simulink model "ctrl_ez"  (R2024b)
settings: configuration reference "CONFI" (kept outside this file)
InitFcn:
  | fidelity_pfc_vals;
  | wl=2*pi*50*150e-6;
  | 
  | gain_vac=1/(220*sqrt(2));
  | kpd = 5;
  | kpq = 5;
  | 
  | 
  | kid   =  1e2;
  | kiq   =  1e2;
  | 
  | kpvdc = .3;
  | kivdc =  .001;
values from neighbouring files (symbols this model uses):
  cos_th = cos(2*pi*50*t)    [fidelity_pfc_vals.m]
  sin_th = sin(2*pi*50*t)    [fidelity_pfc_vals.m]
  sin_th_vb = sin((2*pi*50*t)-(2*pi/3))    [fidelity_pfc_vals.m]
  sin_th_vc = sin((2*pi*50*t)+(2*pi/3))    [fidelity_pfc_vals.m]
  ts = 0.0001    [dic_pfc3ph.sldd]    (also in dictionary.sldd)
  tsw = 1/(fsw*1e3)    (= 1.53846153846e-05)    [fidelity_pfc_vals.m]
undefined symbols (not defined in the file or in its folder): DiscIntNeverNeededParam
libraries: mcbcontrolslib x18, simulink x5, dspswit3 x4, simulink_extras x2, slpidlib x2
(part 2 of 2)

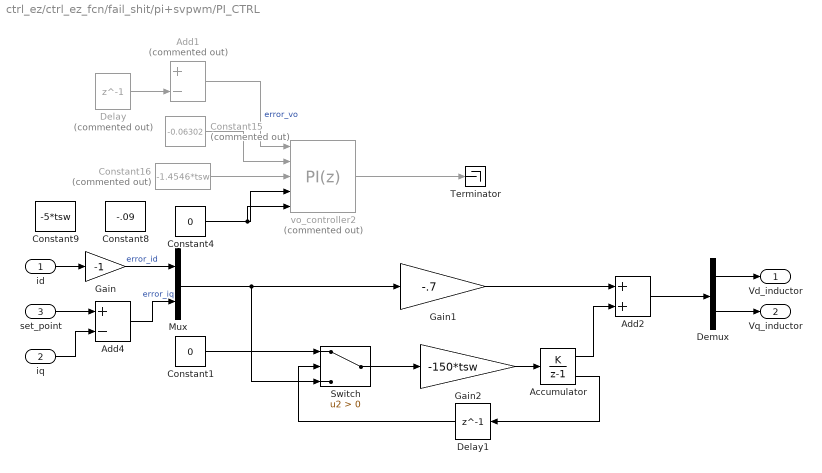
== system ctrl_ez/ctrl_ez_fcn/fail_shit/pi+svpwm/PI_CTRL ==
  id : Inport
  iq : Inport  Port=2  OutDataTypeStr=single
  set_point : Inport  Port=3
  Accumulator : DiscreteIntegrator  IntegratorMethod=Accumulation: Forward Euler  SampleTime=-1  LimitOutput=on  UpperSaturationLimit=50  LowerSaturationLimit=-50  ShowSaturationPort=on  ICPrevOutput=DiscIntNeverNeededParam  ICPrevScaledInput=DiscIntNeverNeededParam
  Add1 : Sum  Commented=on  Inputs=+-
  Add2 : Sum
  Add4 : Sum  Inputs=+-
  Constant1 : Constant  Value=0  OutDataTypeStr=single  SampleTime=-1
  Constant15 : Constant  Commented=on  Value=-0.06302  OutDataTypeStr=single  SampleTime=-1
  Constant16 : Constant  Commented=on  Value=-1.4546*tsw  OutDataTypeStr=single  SampleTime=-1
  Constant4 : Constant  Value=0  OutDataTypeStr=single  SampleTime=-1
  Constant8 : Constant  Value=-.09  OutDataTypeStr=single  SampleTime=-1
  Constant9 : Constant  Value=-5*tsw  OutDataTypeStr=single  SampleTime=-1
  Delay : Delay  Commented=on  DelayLength=1  InitialCondition=580
  Delay1 : Delay  DelayLength=1  InputProcessing=Columns as channels (frame based)
  Demux : Demux  Outputs=2
  Gain : Gain  Gain=-1  OutDataTypeStr=single
  Gain1 : Gain  Gain=-.7  OutDataTypeStr=single
  Gain2 : Gain  Gain=-150*tsw  OutDataTypeStr=single
  Mux : Mux  Inputs=2
  Switch : Switch  Criteria=u2 > Threshold  SaturateOnIntegerOverflow=off  InputSameDT=off
  Terminator : Terminator
  vo_controller2 : slpidlib/PID Controller  Commented=on  Controller=PI  Form=Parallel  TimeDomain=Discrete-time  UseExternalTs=on  SampleTime=-1  IntegratorMethod=Forward Euler  FilterMethod=Forward Euler  ControllerParametersSource=external  P=-0.053025  I=-1.4546  UseKiTs=on  D=0  UseExternalDerivativeSource=off  N=100  UseFilter=on  TunerSelectOption=Transfer Function Based (PID Tuner App)  InitialConditionSource=external  InitialConditionForIntegrator=0  InitialConditionForFilter=0  DifferentiatorICPrevScaledInput=0  ExternalReset=level  TrackingMode=off  Kt=1  LimitOutput=on  SatLimitsSource=internal  UpperSaturationLimit=300  LowerSaturationLimit=-300  LinearizeAsGain=on  AntiWindupMode=clamping  Kb=1  LimitIntegrator=off  UpperIntegratorSaturationLimit=inf  LowerIntegratorSaturationLimit=-inf  POutMin=[]  POutMax=[]  IOutMin=[]  IOutMax=[]  DOutMin=[]  DOutMax=[]  NOutMin=[]  NOutMax=[]  SumOutMin=[]  SumOutMax=[]  SaturationOutMin=[]  SaturationOutMax=[]  PParamMin=[]  PParamMax=[]  IParamMin=[]  IParamMax=[]  DParamMin=[]  DParamMax=[]  NParamMin=[]  NParamMax=[]  KbParamMin=[]  KbParamMax=[]  KtParamMin=[]  KtParamMax=[]  KbOutMin=[]  KbOutMax=[]  KtOutMin=[]  KtOutMax=[]  IntegratorOutMin=[]  IntegratorOutMax=[]  FilterOutMin=[]  FilterOutMax=[]  SumI1OutMin=[]  SumI1OutMax=[]  SumI2OutMin=[]  SumI2OutMax=[]  SumI3OutMin=[]  SumI3OutMax=[]  SumI4OutMin=[]  SumI4OutMax=[]  SumDOutMin=[]  SumDOutMax=[]  DifferentiatorOutMin=[]  DifferentiatorOutMax=[]  FilterDiffOutCoefMin=[]  FilterDiffOutCoefMax=[]  ReciprocalOutMin=[]  ReciprocalOutMax=[]  SumDenOutMin=[]  SumDenOutMax=[]  SumNumOutMin=[]  SumNumOutMax=[]  DivideOutMin=[]  DivideOutMax=[]  UdiffTsProdOutMin=[]  UdiffTsProdOutMax=[]  NTsProdOutMin=[]  NTsProdOutMax=[]  UintegralTsProdOutMin=[]  UintegralTsProdOutMax=[]  UngainTsProdOutMin=[]  UngainTsProdOutMax=[]  ClampingZeroOutDataTypeStr=Inherit: Inherit via back propagation  ClampingZeroOutMin=[]  ClampingZeroOutMax=[]  FilterDenConstantOutDataTypeStr=Inherit: Inherit via back propagation  FilterDenConstantOutMin=[]  FilterDenConstantOutMax=[]  PCopyOutDataTypeStr=Inherit: Inherit via back propagation  PCopyOutMin=[]  PCopyOutMax=[]  NCopyOutDataTypeStr=Inherit: Inherit via back propagation  NCopyOutMin=[]  NCopyOutMax=[]  IntegratorContinuousStateAttributes=''  IntegratorStateMustResolveToSignalObject=off  IntegratorRTWStateStorageClass=Auto  FilterContinuousStateAttributes=''  FilterStateMustResolveToSignalObject=off  FilterRTWStateStorageClass=Auto  ParallelPVariant=ExternalParameters  IdealPVariant=Disabled  IVariant=ExternalParameters  DVariant=Disabled  IntegratorVariant=Discrete  SatVariant=Enabled  AWVariant=DiscClampingParallel  PCopyVariant=Disabled  TRVariant=Disabled  FdbkBlocksVariant=Forward  IdealPFdbkVariant=Disabled  SatFdbkVariant=Disabled  DerivativeFilterVariant=Disabled  NVariant=Disabled  NCopyVariant=Disabled_SignalSpec  FilterICVariant=Disabled  IntegratorICVariant=ExternalICs  ExternalResetVariant=ExternalReset  TRSumVariant=Passthrough  SumFdbkVariant=Disabled  SumVariant=Sum_PI  TsampFilterVariant=InternalTs  TsampNgainVariant=Passthrough  TsampIntegralVariant=Passthrough  ExternalSaturationOutDataTypeStr=Inherit: Same as second input  DerivativeSourceVariant=Disabled  PreIntVariant=InternalPreInt
  Vd_inductor : Outport
  Vq_inductor : Outport  Port=2
  wires:
  Delay/1 -> Add1/2
  id/1 -> Gain/1
  Gain1/1 -> Add2/1
  set_point/1 -> Add4/1
  iq/1 -> Add4/2
  Demux/1 -> Vd_inductor/1
  Add1/1 -> vo_controller2/1  "error_vo"
  Add4/1 -> Mux/2  "error_iq"
  Add2/1 -> Demux/1
  Gain/1 -> Mux/1  "error_id"
  Constant15/1 -> vo_controller2/2
  Constant16/1 -> vo_controller2/3
  Mux/1 -> Switch/3, Gain1/1
  Constant1/1 -> Switch/1
  vo_controller2/1 -> Terminator/1
  Switch/1 -> Gain2/1
  Delay1/1 -> Switch/2
  Gain2/1 -> Accumulator/1
  Accumulator/1 -> Add2/2
  Accumulator/2 -> Delay1/1
  Demux/2 -> Vq_inductor/1
  Constant4/1 -> vo_controller2/4, vo_controller2/5

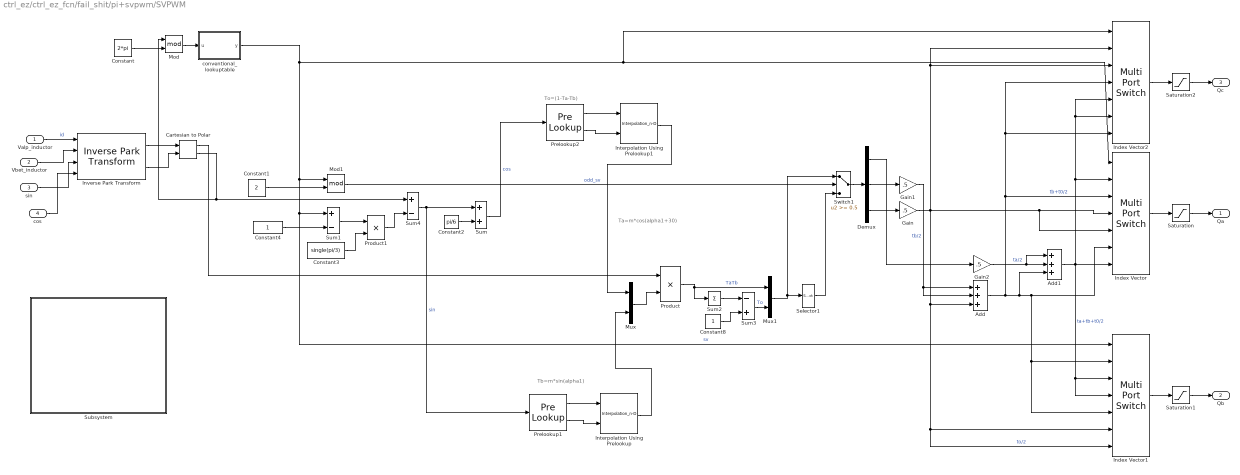
== system ctrl_ez/ctrl_ez_fcn/fail_shit/pi+svpwm/SVPWM ==
  note: Tb=m*sin(alpha1)
  note: Ta=m*cos(alpha1+30)
  note: To=(1-Ta-Tb)
  Valp_inductor : Inport
  Vbet_inductor : Inport  Port=2
  sin : Inport  Port=3
  cos : Inport  Port=4
  Add : Sum  Inputs=+++
  Add1 : Sum  Inputs=+++
  Cartesian to Polar : simulink_extras/Transformations/Cartesian to Polar
  Constant : Constant  Value=2*pi  OutDataTypeStr=single  SampleTime=-1
  Constant1 : Constant  Value=2  OutDataTypeStr=single  SampleTime=-1
  Constant2 : Constant  Value=pi/6  OutDataTypeStr=single  SampleTime=-1
  Constant3 : Constant  Value=single(pi/3)  VectorParams1D=off  OutDataTypeStr=single  SampleTime=-1
  Constant4 : Constant  VectorParams1D=off  OutDataTypeStr=single  SampleTime=-1
  Constant8 : Constant  OutDataTypeStr=single  SampleTime=-1
  Demux : Demux  Outputs=3
  Gain : Gain  Gain=.5  OutDataTypeStr=single
  Gain1 : Gain  Gain=.5  OutDataTypeStr=single
  Gain2 : Gain  Gain=.5  OutDataTypeStr=single
  Index Vector : MultiPortSwitch  Inputs=6  DiagnosticForDefault=None  SaturateOnIntegerOverflow=off  InputSameDT=off
  Index Vector1 : MultiPortSwitch  Inputs=6  DiagnosticForDefault=None  SaturateOnIntegerOverflow=off  InputSameDT=off
  Index Vector2 : MultiPortSwitch  Inputs=6  DiagnosticForDefault=None  SaturateOnIntegerOverflow=off  InputSameDT=off
  Interpolation Using Prelookup : Interpolation_n-D  NumberOfTableDimensions=1  Table=single(sin(0:2*pi/1024:2*pi))  InterpMethod=Flat  RemoveProtectionIndex=on  ValidIndexMayReachLast=on  InternalRulePriority=Speed
      settings: InputPortMap=u0,u1
  Interpolation Using Prelookup1 : Interpolation_n-D  NumberOfTableDimensions=1  Table=single(cos(0:2*pi/1024:2*pi))  InterpMethod=Flat  RemoveProtectionIndex=on  ValidIndexMayReachLast=on  InternalRulePriority=Speed
      settings: InputPortMap=u0,u1
  Inverse Park Transform : mcbcontrolslib/Inverse Park Transform  PhaseInput=Two inputs  AxisAlignment=D-axis  ThetaInput=Sine and Cosine electrical position  AngleInput=Per-unit  N_points=1024
      settings: LibrarySourceBlock=mcbhdllib/Controls/Math Transforms/Inverse Park Transform
  Mod : Math  Operator=mod
  Mod1 : Math  Operator=mod
  Mux : Mux  Inputs=2
  Mux1 : Mux  Inputs=2
  Prelookup1 : PreLookup  BreakpointsData=single((0:2*pi/1024:2*pi))  IndexSearchMethod=Evenly spaced points  BeginIndexSearchUsingPreviousIndexResult=on  UseLastBreakpoint=on
  Prelookup2 : PreLookup  BreakpointsData=single((0:2*pi/1024:2*pi))  IndexSearchMethod=Evenly spaced points  BeginIndexSearchUsingPreviousIndexResult=on  UseLastBreakpoint=on
  Product : Product  SaturateOnIntegerOverflow=on  OutDataTypeStr=Inherit: Same as first input
  Product1 : Product  OutDataTypeStr=single
  Saturation : Saturate  UpperLimit=.98  LowerLimit=.03
  Saturation1 : Saturate  UpperLimit=.98  LowerLimit=.03
  Saturation2 : Saturate  UpperLimit=.98  LowerLimit=.03
  Selector1 : Selector  InputPortWidth=3  IndexOptions=Index vector (dialog)  Indices=[2 1 3]  OutputSizes=1
  Subsystem : Subsystem
  Sum : Sum  SaturateOnIntegerOverflow=on
  Sum1 : Sum  Inputs=+-  OutDataTypeStr=single  AccumDataTypeStr=single
  Sum2 : Sum  Inputs=1  SaturateOnIntegerOverflow=on
  Sum3 : Sum  Inputs=-+  SaturateOnIntegerOverflow=on
  Sum4 : Sum  Inputs=+-  SaturateOnIntegerOverflow=on
  Switch1 : Switch  Threshold=0.5  InputSameDT=off
  conventional_lookuptable : MATLAB Function  TreatAsAtomicUnit=on
  Qa : Outport
  Qb : Outport  Port=2
  Qc : Outport  Port=3
  wires:
  Cartesian to Polar/2 -> Mod/1, Sum4/1
  Demux/2 -> Gain1/1
  Constant/1 -> Mod/2
  Gain1/1 -> Add/1, Add/2  "tb/2"
  Cartesian to Polar/1 -> Product/1
  Constant1/1 -> Mod1/2
  conventional_lookuptable/1(y) -> Index Vector1/1, Sum1/1, Mod1/1, Index Vector2/1, Index Vector/1  "sv"
  Constant4/1 -> Sum1/2
  Mod1/1 -> Switch1/2  "odd_sv"
  Constant3/1 -> Product1/2
  Constant2/1 -> Sum/2
  Demux/1 -> Gain2/1
  Sum4/1 -> Prelookup1/1, Sum/1  "sin"
  Sum/1 -> Prelookup2/1  "cos"
  Mux/1 -> Product/2
  Product/1 -> Mux1/1, Sum2/1  "TaTb"
  Sum2/1 -> Sum3/1
  Constant8/1 -> Sum3/2
  Sum3/1 -> Mux1/2  "To"
  Mux1/1 -> Switch1/1, Selector1/1
  Selector1/1 -> Switch1/3
  Switch1/1 -> Demux/1
  Demux/3 -> Gain/1
  Gain/1 -> Index Vector1/7, Index Vector1/6, Add/3, Index Vector/5, Index Vector/4, Index Vector2/3, Index Vector2/2  "to/2"
  Gain2/1 -> Add1/1, Add1/2  "ta/2"
  Add/1 -> Index Vector1/5, Index Vector1/2, Index Vector/6, Add1/3, Index Vector2/4, Index Vector2/7, Index Vector/3  "tb+t0/2"
  Add1/1 -> Index Vector1/4, Index Vector1/3, Index Vector2/5, Index Vector2/6, Index Vector/2, Index Vector/7  "ta+tb+t0/2"
  Mod/1 -> conventional_lookuptable/1(u)
  Prelookup1/1 -> Interpolation Using Prelookup/1
  Prelookup1/2 -> Interpolation Using Prelookup/2
  Prelookup2/2 -> Interpolation Using Prelookup1/2
  Prelookup2/1 -> Interpolation Using Prelookup1/1
  Interpolation Using Prelookup/1 -> Mux/2
  Interpolation Using Prelookup1/1 -> Mux/1
  Sum1/1 -> Product1/1
  Index Vector2/1 -> Saturation2/1
  Index Vector/1 -> Saturation/1
  Index Vector1/1 -> Saturation1/1
  Product1/1 -> Sum4/2
  Saturation2/1 -> Qc/1
  Saturation/1 -> Qa/1
  Saturation1/1 -> Qb/1
  Valp_inductor/1 -> Inverse Park Transform/1  "id"
  Vbet_inductor/1 -> Inverse Park Transform/2
  Inverse Park Transform/2 -> Cartesian to Polar/2
  Inverse Park Transform/1 -> Cartesian to Polar/1
  sin/1 -> Inverse Park Transform/3
  cos/1 -> Inverse Park Transform/4

== system ctrl_ez/ctrl_ez_fcn/fail_shit/pi+svpwm/clarke_park_tf ==
  a : Inport
  b : Inport  Port=2
  c : Inport  Port=3
  sin : Inport  Port=4
  cos : Inport  Port=5
  Clarke Transform : mcbcontrolslib/Clarke Transform  VariantControl=Variant2  PhaseInput=Three inputs  EnPowerInv=off
      settings: LibrarySourceBlock=mcbhdllib/Controls/Math Transforms/Clarke Transform
  Demux : Demux  Outputs=3
  Mux : Mux  Inputs=3
  Park Transform : mcbcontrolslib/Park Transform  PhaseInput=Two inputs  AxisAlignment=D-axis  ThetaInput=Sine and Cosine electrical position  AngleInput=Per-unit  N_points=1024
      settings: LibrarySourceBlock=mcbhdllib/Controls/Math Transforms/Park Transform
  Terminator : Terminator
  id : Outport
  iq : Outport  Port=2
  wires:
  a/1 -> Mux/1
  b/1 -> Mux/2
  c/1 -> Mux/3
  Mux/1 -> Clarke Transform/1
  Clarke Transform/1 -> Demux/1
  Demux/1 -> Park Transform/1
  Demux/3 -> Terminator/1
  Demux/2 -> Park Transform/2
  cos/1 -> Park Transform/4
  sin/1 -> Park Transform/3
  Park Transform/1 -> id/1
  Park Transform/2 -> iq/1

== system ctrl_ez/ctrl_ez_fcn/fail_shit/pi+svpwm/svm ==
  note: (Vmin+Vmax)/2
  In1 : Inport
  In2 : Inport  Port=2
  In3 : Inport  Port=3
  Add : Sum  Inputs=+-  RndMeth=Simplest  OutDataTypeStr=Inherit: Same as first input
  Add1 : Sum  Inputs=+-  RndMeth=Simplest  OutDataTypeStr=Inherit: Same as first input
  Add2 : Sum  RndMeth=Simplest  OutDataTypeStr=Inherit: Same as first input
  Add3 : Sum  RndMeth=Simplest  OutDataTypeStr=Inherit: Same as first input
  Add4 : Sum  RndMeth=Simplest  OutDataTypeStr=Inherit: Same as first input
  Add5 : Sum  Inputs=+-  RndMeth=Simplest  OutDataTypeStr=Inherit: Same as first input
  Demux : Demux  Outputs=3
  Demux1 : Demux  Outputs=3
  Demux2 : Demux  Outputs=3
  Gain : Gain  Gain=2/sqrt(3)  RndMeth=Simplest  OutDataTypeStr=Inherit: Same as input  ParamDataTypeStr=Inherit: Same as input
  Max : MinMax  Function=max  Inputs=3  RndMeth=Simplest  OutDataTypeStr=Inherit: Same as first input
  Min : MinMax  Inputs=3  RndMeth=Simplest  OutDataTypeStr=Inherit: Same as first input
  Min1 : MinMax  Inputs=3  RndMeth=Simplest  OutDataTypeStr=Inherit: Same as first input
  Mux2 : Mux  Inputs=3
  one_by_two : Gain  Gain=.5  RndMeth=Simplest  OutDataTypeStr=Inherit: Same as input  ParamDataTypeStr=Inherit: Same as input
  Out1 : Outport
  wires:
  Gain/1 -> Out1/1
  Add5/1 -> Add3/1, Add4/2, Add2/2
  Demux1/2 -> Add2/1, Min1/2
  Add3/1 -> Mux2/3
  Mux2/1 -> Gain/1
  Demux1/1 -> Add4/1, Min1/3
  Add2/1 -> Mux2/2
  Add4/1 -> Mux2/1
  Demux1/3 -> Min1/1, Add3/2
  Add/1 -> Add1/2  "vmx-vmn"
  Demux/3 -> Max/3
  Demux2/2 -> Min/2
  Demux/2 -> Max/2
  Demux/1 -> Max/1
  Demux2/1 -> Min/1
  Min/1 -> Add/2
  Max/1 -> Add/1
  Demux2/3 -> Min/3
  In1/1 -> Demux2/1, Demux/1, Demux1/1
  Add1/1 -> one_by_two/1  "vdc-vmx+mn"
  In2/1 -> Add1/1
  one_by_two/1 -> Add5/1
  Min1/1 -> Add5/2

== system ctrl_ez/ctrl_ez_fcn/fail_shit/pi+svpwm1/I_SET_PI_CTRL ==
  v_dc_error : Inport  OutDataTypeStr=single
  Accumulator : DiscreteIntegrator  IntegratorMethod=Accumulation: Forward Euler  SampleTime=-1  LimitOutput=on  UpperSaturationLimit=50  LowerSaturationLimit=-50  ShowSaturationPort=on  ICPrevOutput=DiscIntNeverNeededParam  ICPrevScaledInput=DiscIntNeverNeededParam
  Add2 : Sum
  Constant1 : Constant  Value=0  OutDataTypeStr=single  SampleTime=-1
  Delay1 : Delay  DelayLength=1  InputProcessing=Columns as channels (frame based)
  Gain1 : Gain  Gain=1/30  OutDataTypeStr=single
  Gain2 : Gain  Gain=0  OutDataTypeStr=single
  Saturation : Saturate  UpperLimit=30  LowerLimit=-30
  Switch : Switch  Criteria=u2 > Threshold  SaturateOnIntegerOverflow=off  InputSameDT=off
  i_set : Outport
  wires:
  Add2/1 -> Saturation/1
  Gain2/1 -> Accumulator/1
  Gain1/1 -> Add2/1
  Delay1/1 -> Switch/2
  Switch/1 -> Gain2/1
  Constant1/1 -> Switch/1
  Accumulator/1 -> Add2/2
  Accumulator/2 -> Delay1/1
  v_dc_error/1 -> Switch/3, Gain1/1  "error"
  Saturation/1 -> i_set/1

== system ctrl_ez/ctrl_ez_fcn/fail_shit/pi+svpwm1/PI_CTRL ==
  i_error : Inport  OutDataTypeStr=single
  Accumulator : DiscreteIntegrator  IntegratorMethod=Accumulation: Forward Euler  SampleTime=-1  LimitOutput=on  UpperSaturationLimit=50  LowerSaturationLimit=-50  ShowSaturationPort=on  ICPrevOutput=DiscIntNeverNeededParam  ICPrevScaledInput=DiscIntNeverNeededParam
  Add2 : Sum
  Constant1 : Constant  Value=0  OutDataTypeStr=single  SampleTime=-1
  Delay1 : Delay  DelayLength=1  InputProcessing=Columns as channels (frame based)
  Gain1 : Gain  Gain=100  OutDataTypeStr=single
  Gain2 : Gain  Gain=0  OutDataTypeStr=single
  Saturation : Saturate  Commented=through  UpperLimit=300  LowerLimit=-300
  Switch : Switch  Criteria=u2 > Threshold  SaturateOnIntegerOverflow=off  InputSameDT=off
  v_ind : Outport
  wires:
  i_error/1 -> Gain1/1, Switch/3  "error"
  Accumulator/2 -> Delay1/1
  Accumulator/1 -> Add2/2
  Constant1/1 -> Switch/1
  Switch/1 -> Gain2/1
  Delay1/1 -> Switch/2
  Gain1/1 -> Add2/1
  Gain2/1 -> Accumulator/1
  Add2/1 -> Saturation/1
  Saturation/1 -> v_ind/1

== system ctrl_ez/ctrl_ez_fcn/fail_shit/pi+svpwm1/Subsystem ==
  Constant : Constant  Value=0  SampleTime=-1
  Counter : dspswit3/Counter  Direction=Up  CountEvent=Free running  CounterSize=User defined  MaxCount=length(t)  InitialCount=0  Output=Count  HitValue=32  ResetInput=on  SamplesPerFrame=1  Ts=-1  CntDtype=uint32  HitDtype=Logical
  va_lt : LookupNDDirect  NumberOfTableDimensions=1  Table=single(sin_th*230*sqrt(2));  RemoveProtectionInput=on  TableDataTypeStr=single
  vb_lt : LookupNDDirect  NumberOfTableDimensions=1  Table=single(sin_th_vb*230*sqrt(2));  RemoveProtectionInput=on  TableDataTypeStr=single
  vc_lt : LookupNDDirect  NumberOfTableDimensions=1  Table=single(sin_th_vc*230*sqrt(2));  RemoveProtectionInput=on  TableDataTypeStr=single
  angle_wt : Outport
  angle_wt1 : Outport  Port=2
  angle_wt2 : Outport  Port=3
  wires:
  vc_lt/1 -> angle_wt2/1  "angle_wt"
  Counter/1 -> va_lt/1, vc_lt/1, vb_lt/1  "cnt"
  vb_lt/1 -> angle_wt1/1  "angle_wt"
  Constant/1 -> Counter/1
  va_lt/1 -> angle_wt/1  "angle_wt"

== system ctrl_ez/ctrl_ez_fcn/pll/dummy_pll/zcd ==
  v_ac : Inport  OutDataTypeStr=single
  AND : Logic  Inputs=4  AllPortsSameDT=off  OutDataTypeStr=boolean
  Compare To Zero : simulink/Logic and Bit Operations/Compare To Zero  relop=<  OutDataTypeStr=boolean
  Compare To Zero1 : simulink/Logic and Bit Operations/Compare To Zero  relop=<  OutDataTypeStr=boolean
  Compare To Zero2 : simulink/Logic and Bit Operations/Compare To Zero  relop=>  OutDataTypeStr=boolean
  Compare To Zero3 : simulink/Logic and Bit Operations/Compare To Zero  relop=>  OutDataTypeStr=boolean
  Delay : Delay  DelayLength=4
  Delay1 : Delay  DelayLength=1
  Delay2 : Delay  DelayLength=0
  Delay3 : Delay  DelayLength=5
  zcd : Outport
  wires:
  v_ac/1 -> Delay2/1
  Delay3/1 -> Compare To Zero/1
  Delay/1 -> Delay3/1, Compare To Zero1/1
  Delay2/1 -> Compare To Zero3/1, Delay1/1
  Delay1/1 -> Compare To Zero2/1, Delay/1
  Compare To Zero3/1 -> AND/1
  Compare To Zero1/1 -> AND/3
  Compare To Zero/1 -> AND/4
  Compare To Zero2/1 -> AND/2
  AND/1 -> zcd/1

== system ctrl_ez/ctrl_ez_fcn/pll/srf_pll_dco/2nd_lp_filter ==
  u : Inport
  Constant1 : Constant  Value=0  OutDataTypeStr=single  SampleTime=-1
  Constant2 : Constant  Value=2*pi*50  OutDataTypeStr=single  SampleTime=-1
  Gain1 : Gain  Gain=single(2*1/100)
  Integrator : DiscreteIntegrator  IntegratorMethod=Accumulation: Forward Euler  gainval=1/8e3  InitialConditionSource=external  SampleTime=-1  ICPrevOutput=DiscIntNeverNeededParam  ICPrevScaledInput=DiscIntNeverNeededParam
  Integrator1 : DiscreteIntegrator  IntegratorMethod=Accumulation: Forward Euler  gainval=1/8e3  InitialConditionSource=external  SampleTime=-1  ICPrevOutput=DiscIntNeverNeededParam  ICPrevScaledInput=DiscIntNeverNeededParam
  MATLAB Function : MATLAB Function  TreatAsAtomicUnit=on
  Product : Product
  Sum : Sum  Inputs=+--
  y : Outport  VectorParamsAs1DForOutWhenUnconnected=off
  wires:
  Sum/1 -> Product/2
  Constant2/1 -> Integrator1/2
  Constant1/1 -> Integrator/2
  Integrator/1 -> Integrator1/1, Gain1/1
  u/1 -> Sum/1
  Product/1 -> Integrator/1
  Gain1/1 -> Sum/3
  MATLAB Function/1(forward_gain) -> Product/1
  Integrator1/1 -> MATLAB Function/1(Ts), y/1, Sum/2

== system ctrl_ez/ctrl_ez_fcn/ctrl/svm/pi+svpwm1/I_SET_PI_CTRL ==
  v_dc_error : Inport  OutDataTypeStr=single
  Accumulator : DiscreteIntegrator  IntegratorMethod=Accumulation: Forward Euler  SampleTime=-1  LimitOutput=on  UpperSaturationLimit=50  LowerSaturationLimit=-50  ShowSaturationPort=on  ICPrevOutput=DiscIntNeverNeededParam  ICPrevScaledInput=DiscIntNeverNeededParam
  Add2 : Sum
  Constant1 : Constant  Value=0  OutDataTypeStr=single  SampleTime=-1
  Delay1 : Delay  DelayLength=1  InputProcessing=Columns as channels (frame based)
  Gain1 : Gain  Gain=1/30  OutDataTypeStr=single
  Gain2 : Gain  Gain=0  OutDataTypeStr=single
  Saturation : Saturate  UpperLimit=30  LowerLimit=-30
  Switch : Switch  Criteria=u2 > Threshold  SaturateOnIntegerOverflow=off  InputSameDT=off
  i_set : Outport
  wires:
  Add2/1 -> Saturation/1
  Gain2/1 -> Accumulator/1
  Gain1/1 -> Add2/1
  Delay1/1 -> Switch/2
  Switch/1 -> Gain2/1
  Constant1/1 -> Switch/1
  Accumulator/1 -> Add2/2
  Accumulator/2 -> Delay1/1
  v_dc_error/1 -> Switch/3, Gain1/1  "error"
  Saturation/1 -> i_set/1

== system ctrl_ez/ctrl_ez_fcn/ctrl/svm/pi+svpwm1/PI_CTRL ==
  i_error : Inport  OutDataTypeStr=single
  Accumulator : DiscreteIntegrator  IntegratorMethod=Accumulation: Forward Euler  SampleTime=-1  LimitOutput=on  UpperSaturationLimit=50  LowerSaturationLimit=-50  ShowSaturationPort=on  ICPrevOutput=DiscIntNeverNeededParam  ICPrevScaledInput=DiscIntNeverNeededParam
  Add2 : Sum
  Constant1 : Constant  Value=0  OutDataTypeStr=single  SampleTime=-1
  Delay1 : Delay  DelayLength=1  InputProcessing=Columns as channels (frame based)
  Gain1 : Gain  Gain=100  OutDataTypeStr=single
  Gain2 : Gain  Gain=0  OutDataTypeStr=single
  Saturation : Saturate  Commented=through  UpperLimit=300  LowerLimit=-300
  Switch : Switch  Criteria=u2 > Threshold  SaturateOnIntegerOverflow=off  InputSameDT=off
  v_ind : Outport
  wires:
  i_error/1 -> Gain1/1, Switch/3  "error"
  Accumulator/2 -> Delay1/1
  Accumulator/1 -> Add2/2
  Constant1/1 -> Switch/1
  Switch/1 -> Gain2/1
  Delay1/1 -> Switch/2
  Gain1/1 -> Add2/1
  Gain2/1 -> Accumulator/1
  Add2/1 -> Saturation/1
  Saturation/1 -> v_ind/1

== system ctrl_ez/ctrl_ez_fcn/ctrl/svm/pi+svpwm1/Subsystem ==
  Constant : Constant  Value=0  SampleTime=-1
  Counter : dspswit3/Counter  Direction=Up  CountEvent=Free running  CounterSize=User defined  MaxCount=length(t)  InitialCount=0  Output=Count  HitValue=32  ResetInput=on  SamplesPerFrame=1  Ts=-1  CntDtype=uint32  HitDtype=Logical
  va_lt : LookupNDDirect  NumberOfTableDimensions=1  Table=single(sin_th*230*sqrt(2));  RemoveProtectionInput=on  TableDataTypeStr=single
  vb_lt : LookupNDDirect  NumberOfTableDimensions=1  Table=single(sin_th_vb*230*sqrt(2));  RemoveProtectionInput=on  TableDataTypeStr=single
  vc_lt : LookupNDDirect  NumberOfTableDimensions=1  Table=single(sin_th_vc*230*sqrt(2));  RemoveProtectionInput=on  TableDataTypeStr=single
  angle_wt : Outport
  angle_wt1 : Outport  Port=2
  angle_wt2 : Outport  Port=3
  wires:
  vc_lt/1 -> angle_wt2/1  "angle_wt"
  Counter/1 -> va_lt/1, vc_lt/1, vb_lt/1  "cnt"
  vb_lt/1 -> angle_wt1/1  "angle_wt"
  Constant/1 -> Counter/1
  va_lt/1 -> angle_wt/1  "angle_wt"

== system ctrl_ez/ctrl_ez_fcn/fail_shit/pi+svpwm/SVPWM/Subsystem ==
  note: Three-Phase VSC Diagram
  note: U7 = 1 1 1
  note: --------------------------------------------------------
  note: Q1 Q3 Q5
  note: -
  note: |
      | |
      | |
  note: |
      | |
      | |
      | |
      | |
      | |
  note: [Q6]
  note: [Q5]
  note: [Q4]
  note: [Q3]
  note: U3 = 0 1 0
  note: ---Va
  note: U5 = 0 0 1
  note: Vdc
  note: [5]
  note: 3                       2
      |       3                   2
      |         3               2
      |           3           2
      |             3       2
      |               3   2
      | 4 4 4 4 4 4 4 4 0 1 1 1 1 1 1 1 1
      |               5   6
      |             5       6
      |           5           6
      |         5               6
      |       5                   6
      |     5                       6
  note: |
      | |
      | |
  note: |
      | |
      | |
  note: [2]
  note: U4 = 0 1 1
  note: U6 = 1 0 1
  note: [3]
  note: [1]
  note: [6]
  note: |
      | |
      | |
  note: |
      | |
      | |
      | |
      | |
      | |
  note: U1 = 1 0 0
  note: [n] = Sector number
  note: [Q1]
  note: U2 = 1 1 0
  note: [Q2]
  note: ---Vc
  note: U0 = 0 0 0
  note: |
      | |
      | |
  note: [4]
  note: |
      | |
      | |
  note: --------------------------------------------------------
  note: ---Vb
  note: +
  note: |
      | |
      | |
      | |
      | |
      | |
  INFO : Subsystem
      mask Display: disp('?')

== system ctrl_ez/ctrl_ez_fcn/fail_shit/pi+svpwm/SVPWM/Subsystem/INFO ==
  note: Pattern #2:
      | With this pattern, identified as "Hardware-Determined" by Texas Instruments, there is always one PWM channel staying constant for the entire PWM period.
      |  So the number of switching times for this pattern is less than pattern #1. As a result, switching losses will be reduced with Pattern #2.
  note: Pattern #1:
      | With this pattern, identified as "Software-Determined" by Texas Instruments, each PWM channel switches twice per every PWM period.
  note: --------------------------------------------------------------------------------------------------------------------------------------------------------------------
  note: Reference: Application Report SPRA524
      | Space-Vector PWM with TMS320C24x Using H/W & S/W Determined Switching Patterns
      | Zhenyu Yu, Texas Instruments
  note: The objective of the SV PWM technique is to approximate the reference voltage vector (U*) instantaneously
      | by combination of the switching states corresponding to the basic space vectors.
  note: U7 = 1 1 1
  note: Q1 Q3 Q5
  note: --------------------------------------------------------
  note: Three-Phase VSC Diagram
  note: -
  note: +
  note: --------------------------------------------------------
  note: |
      | |
      | |
  note: ---Vc
  note: |
      | |
      | |
  note: |
      | |
      | |
      | |
      | |
      | |
  note: [Q6]
  note: [Q5]
  note: |
      | |
      | |
  note: ---Vb
  note: |
      | |
      | |
  note: |
      | |
      | |
      | |
      | |
      | |
  note: [Q4]
  note: [Q3]
  note: |
      | |
      | |
  note: ---Va
  note: |
      | |
      | |
  note: |
      | |
      | |
      | |
      | |
      | |
  note: [Q2]
  note: [Q1]
  note: Vdc
  note: [n] = Sector number
  note: [2]
  note: Basic Space Vectors and Switching States
  note: U4 = 0 1 1
  note: U5 = 0 0 1
  note: U6 = 1 0 1
  note: U0 = 0 0 0
  note: U3 = 0 1 0
  note: U2 = 1 1 0
  note: U1 = 1 0 0
  note: [6]
  note: [5]
  note: [4]
  note: [3]
  note: [1]
  note: 3                       2
      |       3                   2
      |         3               2
      |           3           2
      |             3       2
      |               3   2
      | 4 4 4 4 4 4 4 4 0 1 1 1 1 1 1 1 1
      |               5   6
      |             5       6
      |           5           6
      |         5               6
      |       5                   6
      |     5                       6
  note: Two symmetrical switching patterns have been implemented:

== matlab function ctrl_ez/ctrl_ez_fcn/pll/SC/sum ==
  data: a input; c output; b input
function c = fcn(a,b)

c=(a-b);
end

== matlab function ctrl_ez/ctrl_ez_fcn/pll/SC/sum1 ==
  data: a input; c output; b input
function c = fcn(a,b)

c=(a-b);
end

== matlab function ctrl_ez/ctrl_ez_fcn/pll/srf_pll_dco/dco ==
  data: cos_th_1 input single; sin_th_1 input single; th_1 input single; th output single; sin_th output single; wo input single; cos_th output single
function [th,sin_th,cos_th]= dco(cos_th_1,sin_th_1,th_1,wo)
        % ws=(2*pi*50);
        wout=(wo);
        tsample=single(1/8e3);
        %Sin is for showing the overlaping w the input 
        sin_th=sin_th_1+(cos_th_1*wout*tsample); %Sin(t+dt)=sin(t)+cos(t)*dt
        cos_th=cos_th_1-(sin_th_1*wout*tsample);
        
        sin_th=max([sin_th -1]);
        cos_th=max([cos_th -1]);

        sin_th=min([sin_th 1]);
        cos_th=min([cos_th 1]);

        th=th_1+(wout*tsample);

        if sin_th>=0 && sin_th_1<=0
            th=single(0);    %fi(pi,1,32,29); %zero crossing reseting phase angle
        end
      
end

== matlab function ctrl_ez/ctrl_ez_fcn/ctrl/svm/section_cal/sector_selection ==
  data: u input single; aw_ input; y output single; alpha output; oddsect output; theta output; u2 input
function [y,alpha,oddsect,theta] = fcn(u,aw_, u2)
%%
% if aw_<u2
    theta=u2-pi;
% else    
    theta=single(pi)+u2;
    if theta<0
      theta=single(pi)+u2;      
    end
% end
%%





    if (u>=single(0) && u<single(pi/3))
         %sector 1
         y=single(0);
         oddsect=true;        
    elseif u>=single(pi/3) && u<single(2*pi/3)
         %sector 2
         y=single(1);
         oddsect = false;           
    elseif  u>=single(2*pi/3) && u<single(pi)
        %sector 3
         y=single(2);
         oddsect=true;       
    elseif u>=single(pi) && u<single(4*pi/3)
        %sector 4
        y=single(3);
        oddsect = false;
    elseif u>=single(4*pi/3) && u<single(5*pi/3)
        %sector 5
        y=single(4); 
        oddsect=true;
    elseif u>=single(5*pi/3) && u<single(2*pi)
        %sector 6
        y=single(5);
        oddsect = false; 
    % elseif u>=single(11*pi/6) && u<=single(2*pi)
    %     %sector 5.0 
    %     y=single(4);
    %        oddsect=true;
    else
        y=single(1);
        oddsect = false;
    end
    alpha = u - (y*single(pi/3));



%% 
    % if (u>=single(0) && u<single(pi/6))
    %      %sector 5
    %      y=single(4);
    %      oddsect=true;
    %      alpha = u + (single(pi/6));
    % elseif u>=single(pi/6) && u<single(pi/2)
    %      %sector 6
    %        y=single(5);
    %        oddsect = false;
    %        alpha = u - (single(pi/6));
    % elseif  u>=single(pi/2) && u<single(5*pi/6)
    %     %sector 1
    %        y=single(0);
    %        oddsect=true;
    %        alpha = u - (single(pi/2));
    % elseif u>=single(5*pi/6) && u<single(7*pi/6)
    %     %sector 2
    %        y=single(1);
    %        oddsect = false;
    %        alpha = u - (5*single(pi/6));
    % elseif u>=single(7*pi/6) && u<single(3*pi/2)
    %     %sector 3
    %        y=single(2); 
    %        oddsect=true;
    %        alpha = u - (single(7*pi/6));
    % elseif u>=single(3*pi/2) && u<single(11*pi/6)
    %     %sector 4
    %        y=single(3);
    %        oddsect = false; 
    %        alpha = u - (3*single(pi/2));
    % elseif u>=single(11*pi/6) && u<=single(2*pi)
    %     %sector 5.0 
    %     y=single(4);
    %        oddsect=true;
    %     alpha = u - (11*single(pi/6));
    % else
    %     y=single(1);
    %     alpha = single(0);
    %     oddsect = false;
    % end

end

== matlab function ctrl_ez/ctrl_ez_fcn/vd_vq/park_tf ==
  data: vd_park output; vp_alpha input; vq_park output; vp_betha input; sin_th_k_1 input; cos_th_k_1 input
  function [vd_park,vq_park] = park(vp_alpha,vp_betha,sin_th_k_1,cos_th_k_1)

vq_park=(sin_th_k_1*vp_betha+cos_th_k_1*vp_alpha);%(-sin_th_k_1*vp_alpha+cos_th_k_1*vp_betha);
vd_park=(sin_th_k_1*vp_alpha-cos_th_k_1*vp_betha);




end

== matlab function ctrl_ez/ctrl_ez_fcn/pll/srf_pll_dco/pi_ctrl ==
  data: vq_park input single; w_pi output single; vq_park_k_1 input single; w_pi_k_1 input single
function w_pi = pi_ctrl(vq_park,vq_park_k_1,w_pi_k_1)

fs=single(8e3);
ts=1/fs;
wn_pi=single(100*2*pi);%200*2*pi; 
sig_pi=single(.3);%.05;
vac_peak_pi=single(3*3.3);

kp = single(2*wn_pi*sig_pi/vac_peak_pi);
ki = single(2*vac_peak_pi/(4*sig_pi*sig_pi));

pi_n1=kp;
pi_n2=(ki*ts)-kp;
sat=single(285);
w_pi=((vq_park)*pi_n1+(vq_park_k_1)*pi_n2+w_pi_k_1);

% 
% if (w_pi*40)>single(sat*2*pi)
%     w_pi=single(2*85*pi);
% end
% if (w_pi*40)<single(-sat*2*pi)
%     w_pi=single(-2*85*pi);
% end

end

== matlab function ctrl_ez/ctrl_ez_fcn/fail_shit/pi+svpwm/SVPWM/conventional_lookuptable ==
  data: u input single; y output single
function y = fcn(u)

switch u
    % case u>=single(0) && u<single(pi/3)
    %     y=single(1);
    % case u>=single(pi/3) && u<single(2*pi/3)
    %     y=single(2);
    % case u>=single(2*pi/3) && u<single(pi)
    %     y=single(3);
    % case u>=single(pi) && u<single(4*pi/3)
    %     y=single(4);
    % case u>=single(4*pi/3) && u<single(5*pi/3)
    %     y=single(5);
    % case u>=single(5*pi/3) && u<single(2*pi)
    %     y=single(6);        
    % otherwise
    %     y=single(1);
    case u<single(pi/3)
        y=single(1);
    case u<single(2*pi/3)
        y=single(2);
    case u<single(pi)
        y=single(3);
    case u<single(4*pi/3)
        y=single(4);
    case u<single(5*pi/3)
        y=single(5);
    case u<single(2*pi)
        y=single(6);        
    otherwise
        y=single(1);


end

== matlab function ctrl_ez/ctrl_ez_fcn/ctrl/id_iq/park_tf ==
  data: vd_park output; vp_alpha input; vq_park output; vp_betha input; sin_th_k_1 input; cos_th_k_1 input
  function [vd_park,vq_park] = park(vp_alpha,vp_betha,sin_th_k_1,cos_th_k_1)

vq_park=(sin_th_k_1*vp_betha+cos_th_k_1*vp_alpha);     %(-sin_th_k_1*vp_alpha+cos_th_k_1*vp_betha);
vd_park=(sin_th_k_1*vp_alpha-cos_th_k_1*vp_betha);




end

== matlab function ctrl_ez/ctrl_ez_fcn/ctrl/svm/mine_invpark_tf ==
  data: vp_alpha output; vd_park input; vp_betha output; vq_park input; sin_th_k_1 input; cos_th_k_1 input
  function [vp_alpha,vp_betha] = park(vd_park,vq_park,sin_th_k_1,cos_th_k_1)


vp_betha= -(cos_th_k_1*vd_park - sin_th_k_1*vq_park)/(cos_th_k_1^2 + sin_th_k_1^2)
vp_alpha= (cos_th_k_1*vq_park + sin_th_k_1*vd_park)/(cos_th_k_1^2 + sin_th_k_1^2)
% 
% vq_park=(sin_th_k_1*vp_betha+cos_th_k_1*vp_alpha);%(-sin_th_k_1*vp_alpha+cos_th_k_1*vp_betha);
% vd_park=(sin_th_k_1*vp_alpha-cos_th_k_1*vp_betha);




end

== matlab function ctrl_ez/ctrl_ez_fcn/ctrl/svm/section_cal/mod_fcn ==
  data: u input single; y output single
function y  = mod_fcn(u)
   % y = mod(u,single(2*pi));
   y = u - (floor(u/(2*pi))*(2*pi));
end

== matlab function ctrl_ez/ctrl_ez_fcn/pll/pll_lock_subsystem/MATLAB Function ==
  data: u input; y output boolean; cnt_1 input single; cnt output
function [y,cnt] = fcn(u, cnt_1)
y=false;
cnt = cnt_1;
if u == true
   if cnt_1<=single(5*(10e3/50)) 
      cnt = cnt_1 + single(1.0);
      y=false;
   else 
      y=true;
   end
else 
   y=false;
   cnt = single(0.0);
end

== matlab function ctrl_ez/ctrl_ez_fcn/pll/srf_pll_dco/2nd_lp_filter/MATLAB Function ==
  data: Ts input; forward_gain output
function forward_gain  = fcn(Ts)


    forward_gain = single(1/max(Ts,single(1/(100*100))));
   
end

== matlab function ctrl_ez/ctrl_ez_fcn/pll/srf_pll_dco/park_tf ==
  data: vd_park output; vp_alpha input; vq_park output; vp_betha input; sin_th_k_1 input; cos_th_k_1 input
  function [vd_park,vq_park] = park(vp_alpha,vp_betha,sin_th_k_1,cos_th_k_1)

vq_park=(sin_th_k_1*vp_betha)+(cos_th_k_1*vp_alpha);%(-sin_th_k_1*vp_alpha+cos_th_k_1*vp_betha);
vd_park=(sin_th_k_1*vp_alpha)-(cos_th_k_1*vp_betha);




end

== matlab function ctrl_ez/ctrl_ez_fcn/pll/SC/a-b ==
  data: a input; c output; b input
function c = fcn(a,b)

c=0.5*(a-b);
end

== matlab function ctrl_ez/ctrl_ez_fcn/pll/SC/sum2 ==
  data: a input; c output; b input
function c = fcn(a,b)

c=0.5*(a+b);
end
